simulink model "rovSim_trj"  (R2017a)
settings: Solver=ode4  StartTime=0.0  StopTime=10.0  FixedStep=mdl.tStep  RelTol=1e-3
values from neighbouring files (symbols this model uses):
  waypoints = [0,0,0 ... (first row only)    [test_trajectory.m]
undefined symbols (not defined in the file or in its folder): ics, kd, kp, mdl, n_max, rov, Tinv, v_c
settings Model: Creator=e_anderlini  LastModifiedBy=e_anderlini

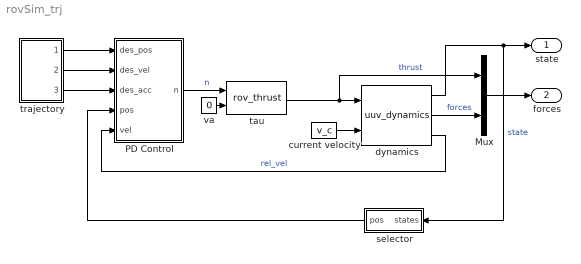
== system rovSim_trj ==
  Mux : Mux  Inputs=[6,18]
  PD Control : Subsystem
  current velocity : Constant  Value=v_c
  dynamics : S-Function  FunctionName=uuv_dynamics  Parameters=rov.weight,rov.buoyancy,rov.G,rov.B,ics,rov.inv_mass',rov.M_A',rov.M_RB',rov.D_L',rov.D_q'  SFunctionDeploymentMode=off  EnableBusSupport=off
  selector : Subsystem
  tau : S-Function  FunctionName=rov_thrust  Parameters=rov.density,rov.prop_diam,rov.K_T,rov.theta,rov.T'  SFunctionDeploymentMode=off  EnableBusSupport=off
  trajectory : Subsystem
  va : Constant  Value=0
  state : Outport
  forces : Outport  Port=2
  wires:
  dynamics/1 -> selector/1(states), state/1  "state"
  tau/1 -> Mux/1, dynamics/1  "thrust"
  Mux/1 -> forces/1
  dynamics/2 -> Mux/2  "forces"
  PD Control/1(n) -> tau/1  "n"
  va/1 -> tau/2
  dynamics/3 -> PD Control/5(vel)  "rel_vel"
  current velocity/1 -> dynamics/2
  selector/1(pos) -> PD Control/4(pos)
  trajectory/1(trj_pos) -> PD Control/1(des_pos)
  trajectory/2(trj_vel) -> PD Control/2(des_vel)
  trajectory/3(trj_acc) -> PD Control/3(des_acc)

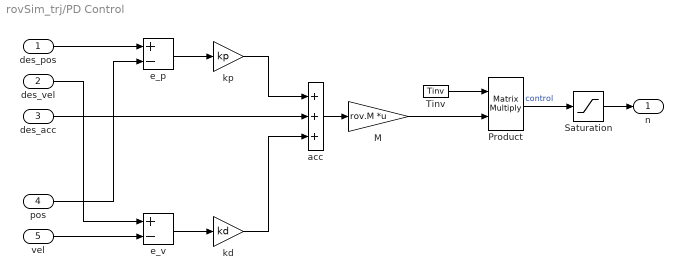
== system rovSim_trj/PD Control ==
  des_pos : Inport
  des_vel : Inport  Port=2
  des_acc : Inport  Port=3
  pos : Inport  Port=4
  vel : Inport  Port=5
  M : Gain  Gain=rov.M  Multiplication=Matrix(K*u)
  Product : Product  Multiplication=Matrix(*)
  Saturation : Saturate  UpperLimit=n_max  LowerLimit=-n_max
  Tinv : Constant  Value=Tinv  VectorParams1D=off
  acc : Sum  Inputs=+++
  e_p : Sum  Inputs=+-
  e_v : Sum  Inputs=+-
  kd : Gain  Gain=kd
  kp : Gain  Gain=kp
  n : Outport
  wires:
  Product/1 -> Saturation/1  "control"
  Tinv/1 -> Product/1
  Saturation/1 -> n/1
  des_pos/1 -> e_p/1
  pos/1 -> e_p/2
  des_vel/1 -> e_v/1
  vel/1 -> e_v/2
  e_p/1 -> kp/1
  e_v/1 -> kd/1
  kp/1 -> acc/1
  des_acc/1 -> acc/2
  kd/1 -> acc/3
  acc/1 -> M/1
  M/1 -> Product/2

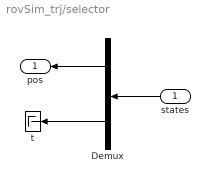
== system rovSim_trj/selector ==
  states : Inport
  Demux : Demux  Outputs=[6,6]
  t : Terminator
  pos : Outport
  wires:
  Demux/1 -> pos/1
  states/1 -> Demux/1
  Demux/2 -> t/1

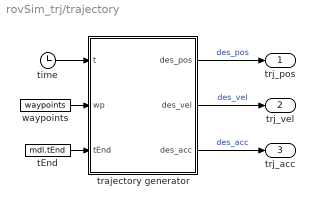
== system rovSim_trj/trajectory ==
  tEnd : Constant  Value=mdl.tEnd
  time : Clock
  trajectory generator : MATLAB Function  TreatAsAtomicUnit=on
  waypoints : Constant  Value=waypoints
  trj_pos : Outport
  trj_vel : Outport  Port=2
  trj_acc : Outport  Port=3
  wires:
  waypoints/1 -> trajectory generator/2(wp)
  trajectory generator/1(des_pos) -> trj_pos/1  "des_pos"
  trajectory generator/2(des_vel) -> trj_vel/1  "des_vel"
  trajectory generator/3(des_acc) -> trj_acc/1  "des_acc"
  tEnd/1 -> trajectory generator/3(tEnd)
  time/1 -> trajectory generator/1(t)

== matlab function rovSim_trj/trajectory/trajectory generator ==
  data: t input; des_pos output; des_vel output; des_acc output; wp input; tEnd input
function [des_pos,des_vel,des_acc] = fcn(t,wp,tEnd)
% fcn.m      e.anderlini@ucl.ac.uk      09/10/2017
%%%%%%%%%%%%%%%%%%%%%%%%%%%%%%%%%%%%%%%%%%%%%%%%%%%%%%%%%%%%%%%%%%%%%%%%%%%
% This function returns the (transverse and angular) acceleration, velocity
% and position of the desired trajectory.
%%%%%%%%%%%%%%%%%%%%%%%%%%%%%%%%%%%%%%%%%%%%%%%%%%%%%%%%%%%%%%%%%%%%%%%%%%%

%% Initialize output size:
des_pos = zeros(6,1);
des_vel = zeros(6,1);
des_acc = zeros(6,1);

%% Define and initialize the desired trajectory:
persistent trj;
if isempty(trj)
    trj = Trajectory('minimum_snap',wp,tEnd);
end

%% Generate the desired trajectory:
trj = trj.trajectory_generation(t);

%% Output the desired data - assume no change in heading for now:
des_pos = [trj.des_pos;zeros(3,1)];
des_vel = [trj.des_vel;zeros(3,1)];
des_acc = [trj.des_acc;zeros(3,1)];

end
